simulink model "Hybrid_Model_PushSum"  (R2016a)
settings: Solver=VariableStepAuto  StartTime=0.0  StopTime=T  RelTol=1e-3
values from neighbouring files (symbols this model uses):
  J = 1500    [run.m]
  number_timers = number_timers_per_node*number_nodes    (= 6)    [run.m]
  number_values = number_values_per_node*number_nodes    (= 12)    [run.m]
  number_values_per_node = 2    [run.m]
  reception_probability = reception_probability_vector(n_probability)    [run.m]
  T = 25    [run.m]
  topology_matrix = squeeze(topology_matrix_matrix(:,:,n_topology))    [run.m]
  type_timer_frequencies = type_timer_frequencies_vector(n_type_timer_frequencies)    [run.m]
  x0 = [2*pi*rand(number_timers,1); values0]    [run.m]
undefined symbols (not defined in the file or in its folder): rule
libraries: simulink x3
settings Model: Creator=Boris  LastModifiedBy=beoro

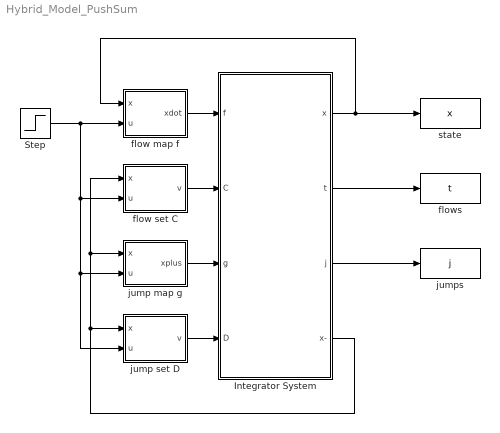
== system Hybrid_Model_PushSum ==
  "Integrator System " : Subsystem
  Step : Step  After=0  SampleTime=0
  flow map f : MATLAB Function  TreatAsAtomicUnit=on
  flow set C : MATLAB Function  TreatAsAtomicUnit=on
  flows : ToWorkspace  VariableName=t  SampleTime=-1
  jump map g : MATLAB Function  Priority=2  TreatAsAtomicUnit=on
  jump set D : MATLAB Function  TreatAsAtomicUnit=on
  jumps : ToWorkspace  VariableName=j  SampleTime=-1
  state : ToWorkspace  VariableName=x  SampleTime=-1
  wires:
  flow map f/1(xdot) -> "Integrator System "/1(f)
  "Integrator System "/4(x-) -> jump map g/1(x), flow set C/1(x), jump set D/1(x)
  "Integrator System "/1(x) -> state/1, flow map f/1(x)
  flow set C/1(v) -> "Integrator System "/2(C)
  "Integrator System "/2(t) -> flows/1
  "Integrator System "/3(j) -> jumps/1
  Step/1 -> flow set C/2(u), jump map g/2(u), jump set D/2(u), flow map f/2(u)
  jump set D/1(v) -> "Integrator System "/4(D)
  jump map g/1(xplus) -> "Integrator System "/3(g)

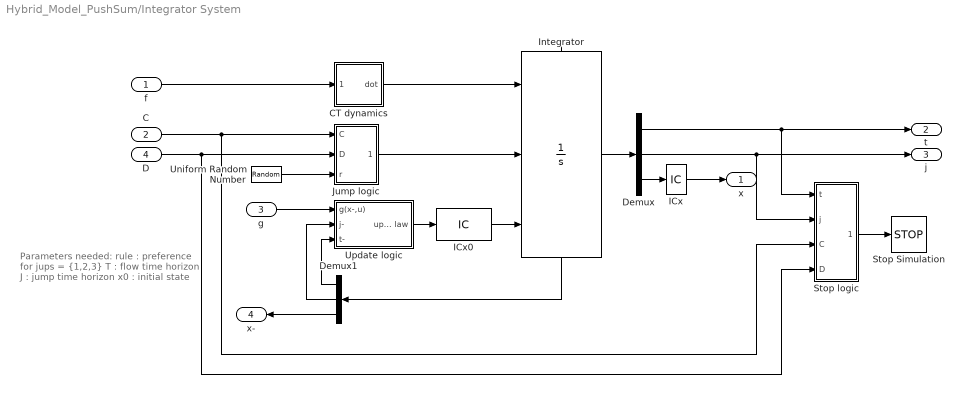
== system Hybrid_Model_PushSum/Integrator System  ==
  note: Parameters needed:
      | rule : preference for jups  = {1,2,3}
      | T    : flow time horizon
      | J     : jump time horizon
      | x0   : initial state
  f : Inport
  C : Inport  Port=2
  g : Inport  Port=3
  D : Inport  Port=4
  CT dynamics : Subsystem
  Demux : Demux  Outputs=[1 1 -1]
  Demux1 : Demux  Outputs=[1 1 -1]
  ICx : InitialCondition  Value=x0
  ICx0 : InitialCondition  Value=[0; 0; x0]
  Integrator : Integrator  ExternalReset=level hold  InitialConditionSource=external  ShowStatePort=on  ZeroCross=off
  Jump logic : Subsystem
  Stop Simulation : Stop
  Stop logic : Subsystem
  Uniform Random Number : UniformRandomNumber  Minimum=0  Seed=abs(floor(100*rand))  SampleTime=0
  Update logic : Subsystem
  x : Outport
  t : Outport  Port=2
  j : Outport  Port=3
  x- : Outport  Port=4
  wires:
  Demux/2 -> j/1, Stop logic/2(j)
  ICx/1 -> x/1
  D/1 -> Jump logic/2(D), Stop logic/4(D)
  Integrator/State -> Demux1/1
  Update logic/1(update law) -> ICx0/1
  ICx0/1 -> Integrator/3
  Jump logic/1(jump) -> Integrator/2
  Demux1/3 -> x-/1
  Demux1/1 -> Update logic/3(t-)
  Stop logic/1(stop) -> Stop Simulation/1
  Demux1/2 -> Update logic/2(j-)
  Integrator/1 -> Demux/1
  CT dynamics/1(dot) -> Integrator/1
  Demux/1 -> t/1, Stop logic/1(t)
  f/1 -> CT dynamics/1(f(x,u))
  g/1 -> Update logic/1(g(x-,u))
  Uniform Random Number/1 -> Jump logic/3(r)
  C/1 -> Jump logic/1(C), Stop logic/3(C)
  Demux/3 -> ICx/1

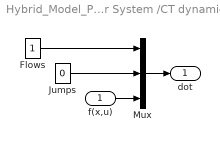
== system Hybrid_Model_PushSum/Integrator System /CT dynamics ==
  f(x,u) : Inport
  Flows : Constant
  Jumps : Constant  Value=0
  Mux : Mux  Inputs=[1 1 -1]
  dot : Outport
  wires:
  f(x,u)/1 -> Mux/3
  Mux/1 -> dot/1
  Flows/1 -> Mux/1
  Jumps/1 -> Mux/2

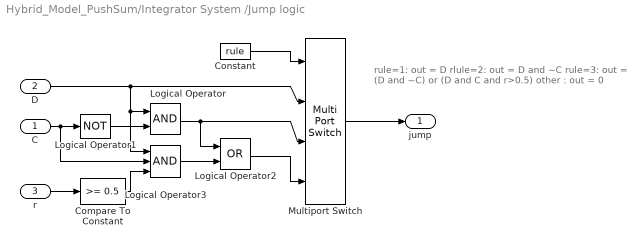
== system Hybrid_Model_PushSum/Integrator System /Jump logic ==
  note: rule=1:  out = D
      | rlule=2: out = D and ~C
      | rule=3:  out = (D and ~C)  or (D and C and r>0.5)
      | other :  out = 0
  C : Inport
  D : Inport  Port=2
  r : Inport  Port=3
  Compare To Constant : simulink/Logic and Bit Operations/Compare To Constant  relop=>=  const=0.5  OutDataTypeStr=uint8
  Constant : Constant  Value=rule
  Logical Operator : Logic  AllPortsSameDT=off  OutDataTypeStr=boolean
  Logical Operator1 : Logic  Operator=NOT  Inputs=1  AllPortsSameDT=off  OutDataTypeStr=boolean
  Logical Operator2 : Logic  Operator=OR  AllPortsSameDT=off  OutDataTypeStr=boolean
  Logical Operator3 : Logic  Inputs=3  AllPortsSameDT=off  OutDataTypeStr=boolean
  Multiport Switch : MultiPortSwitch
  jump : Outport
  wires:
  Logical Operator3/1 -> Logical Operator2/2
  Compare To Constant/1 -> Logical Operator3/3
  Multiport Switch/1 -> jump/1
  Logical Operator2/1 -> Multiport Switch/4
  Logical Operator/1 -> Logical Operator2/1, Multiport Switch/3
  Logical Operator1/1 -> Logical Operator/2
  C/1 -> Logical Operator1/1, Logical Operator3/2
  r/1 -> Compare To Constant/1
  D/1 -> Multiport Switch/2, Logical Operator/1, Logical Operator3/1
  Constant/1 -> Multiport Switch/1

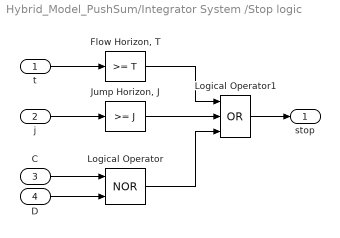
== system Hybrid_Model_PushSum/Integrator System /Stop logic ==
  t : Inport
  j : Inport  Port=2
  C : Inport  Port=3
  D : Inport  Port=4
  "Flow Horizon, T" : simulink/Logic and Bit Operations/Compare To Constant  relop=>=  const=T  OutDataTypeStr=uint8  ZeroCross=off
  "Jump Horizon, J" : simulink/Logic and Bit Operations/Compare To Constant  relop=>=  const=J  OutDataTypeStr=uint8  ZeroCross=off
  Logical Operator : Logic  Operator=NOR  AllPortsSameDT=off  OutDataTypeStr=boolean
  Logical Operator1 : Logic  Operator=OR  Inputs=3  AllPortsSameDT=off  OutDataTypeStr=boolean
  stop : Outport
  wires:
  Logical Operator1/1 -> stop/1
  C/1 -> Logical Operator/1
  j/1 -> "Jump Horizon, J"/1
  t/1 -> "Flow Horizon, T"/1
  D/1 -> Logical Operator/2
  Logical Operator/1 -> Logical Operator1/3
  "Jump Horizon, J"/1 -> Logical Operator1/2
  "Flow Horizon, T"/1 -> Logical Operator1/1

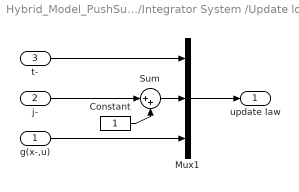
== system Hybrid_Model_PushSum/Integrator System /Update logic ==
  g(x-,u) : Inport
  j- : Inport  Port=2
  t- : Inport  Port=3
  Constant : Constant
  Mux1 : Mux  Inputs=[1 1 -1]
  Sum : Sum  Inputs=|++
  update law : Outport
  wires:
  Constant/1 -> Sum/2
  t-/1 -> Mux1/1
  g(x-,u)/1 -> Mux1/3
  j-/1 -> Sum/1
  Mux1/1 -> update law/1
  Sum/1 -> Mux1/2

== matlab function Hybrid_Model_PushSum/jump set D ==
  data: x input; v output; u input; number_timers parameter
function v  = D(x, u, number_timers) 

%%%%%%%%%%%%%%%%%%%%%%%%%%%%%%%%%%%%%%%%%%%%%%%%%%%%%%%%%%%%%%%%%%%%%%%%%%%
% Matlab Function  Author: Ricardo Sanfelice 
% (Revised by Giampiero Campa)
% (Revised by Pablo Nanez)
%
% Name: D.m
%
% Description: Jump set
%
%%%%%%%%%%%%%%%%%%%%%%%%%%%%%%%%%%%%%%%%%%%%%%%%%%%%%%%%%%%%%%%%%%%%%%%%%%%

    %Jump set:
    v = 0;
    for i = (1:number_timers)
        if ( 2*pi <= x(i) )  %jump condition
            v = 1;           %report jump
        end
    end

end

== matlab function Hybrid_Model_PushSum/flow map f ==
  data: x input; u input; number_timers parameter; xdot output; number_values parameter; type_timer_frequencies parameter

function xdot = f(x, u, number_timers, number_values, type_timer_frequencies)

%%%%%%%%%%%%%%%%%%%%%%%%%%%%%%%%%%%%%%%%%%%%%%%%%%%%%%%%%%%%%%%%%%%%%%%%%%%
% Matlab Function  Author: Ricardo Sanfelice 
% (Revised by Giampiero Campa)
% (Revised by Pablo Nanez)
%
% Name: f.m
%
% Description: Flow map
%
%%%%%%%%%%%%%%%%%%%%%%%%%%%%%%%%%%%%%%%%%%%%%%%%%%%%%%%%%%%%%%%%%%%%%%%%%%%
    
    %User can define other frequencies!!!:
    if(type_timer_frequencies == 1)
        timer_frequencies = 2*pi*ones(number_timers,1);
    end
    if(type_timer_frequencies == 2)
        timer_frequencies = 2*pi*ones(number_timers,1) + 0.1*2*pi*rand(number_timers,1);
    end
    if(type_timer_frequencies == 3)
        timer_frequencies = (2*pi:    pi:  7*pi)' + 0.1*2*pi*rand(number_timers,1);
    end
    if(type_timer_frequencies == 4)
        timer_frequencies = (7*pi:   -pi:  2*pi)' + 0.1*2*pi*rand(number_timers,1);
    end

    %Flow map:
    xdot  = [timer_frequencies; zeros(number_values,1)];

end

== matlab function Hybrid_Model_PushSum/flow set C ==
  data: x input; v output; u input; number_timers parameter
function v  = C(x, u, number_timers) 

%%%%%%%%%%%%%%%%%%%%%%%%%%%%%%%%%%%%%%%%%%%%%%%%%%%%%%%%%%%%%%%%%%%%%%%%%%%
% Matlab Function  Author: Ricardo Sanfelice 
% (Revised by Giampiero Campa)
% (Revised by Pablo Nanez)
%
% Name: C.m
%
% Description: Flow set
%
%%%%%%%%%%%%%%%%%%%%%%%%%%%%%%%%%%%%%%%%%%%%%%%%%%%%%%%%%%%%%%%%%%%%%%%%%%%

    %Flow set:
    v = 1;
%     for i = (1:number_timers)
%         %Invalid flow condition:
%         if ( (x(i) < 0) || (2*pi < x(i)) )  
%             v = 0; 
%         end
%     end

end

== matlab function Hybrid_Model_PushSum/jump map g ==
  data: x input; xplus output; u input; number_timers parameter; number_values parameter; topology_matrix parameter; number_values_per_node parameter; reception_probability parameter

function xplus = g(x, u, number_timers, number_values, topology_matrix, number_values_per_node, reception_probability)

%%%%%%%%%%%%%%%%%%%%%%%%%%%%%%%%%%%%%%%%%%%%%%%%%%%%%%%%%%%%%%%%%%%%%%%%%%%
% Matlab Function  Author: Ricardo Sanfelice 
% (Revised by Giampiero Campa)
% (Revised by Pablo Nanez)
%
% Name: g.m
%
% Description: Jump map
%
%%%%%%%%%%%%%%%%%%%%%%%%%%%%%%%%%%%%%%%%%%%%%%%%%%%%%%%%%%%%%%%%%%%%%%%%%%%

    coder.extrinsic('wrapTo2Pi');

    %Constants:
    epsilon    = zeros(1,number_timers);
    for j = 1:number_timers
        epsilon(j) = 1/(1+sum(topology_matrix(:,j)));
    end
    
    %State:
    xplus_timers        = x(1:number_timers, 1);
    xplus_values        = x(number_timers+1: number_timers+number_values, 1);
    xplus_values_matrix = reshape(xplus_values,[number_values_per_node, number_timers]);
    
    %Update:
    for i = (1:number_timers)
        if ( 2*pi <= x(i,1) )
            xplus_timers(i,1) = wrapTo2Pi(xplus_timers(i,1));
            %This is the protocol:
            xplus_values_matrix(:,i) = epsilon(i)*xplus_values_matrix(:,i);
            for j = (1:number_timers)
                random_value = rand;
                if random_value < reception_probability
                    xplus_values_matrix(:,j) = xplus_values_matrix(:,j) + topology_matrix(i,j)*xplus_values_matrix(:,i);
                end
            end        
        end
    end
    xplus_values = reshape(xplus_values_matrix,[number_values,1]);
    
%     %Limits:
%     for i = (1:number_timers)
%         if ( 2*pi < xplus_timers(i,1) )
%             xplus_timers(i,1) = 2*pi;
%         end
%         if ( xplus_timers(i,1) < 0 )
%             xplus_timers(i,1) = 0;
%         end
%     end
    
    %Complete state:
    xplus = [xplus_timers; xplus_values];

end
